simulink model "CANTXcommunicationunit_4"  (R2024a)
settings: Solver=VariableStepAuto  StartTime=0.0  StopTime=10.0  RelTol=1e-3
undefined symbols (not defined in the file or in its folder): canChannel
libraries: canlib x3, canmsglib x2
settings Model: DataDictionary=BMS_System_dict1.sldd  Creator=hirah  LastModifiedBy=hirah

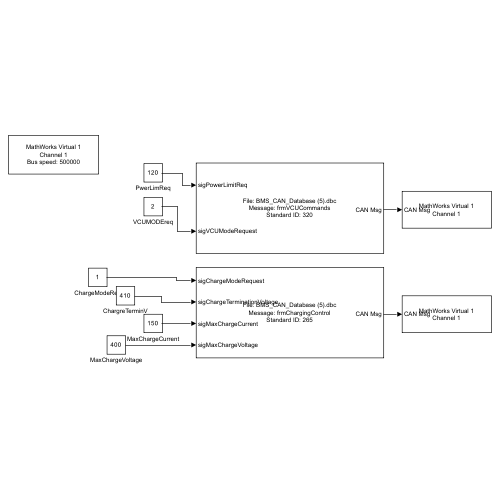
[thumbnail: Simulink's stored preview of the top-level diagram]
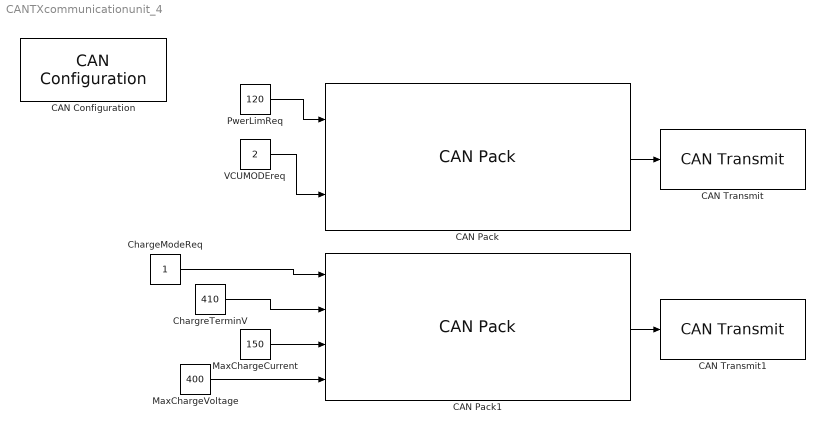
== system CANTXcommunicationunit_4 ==
  CAN Configuration : canlib/CAN Configuration  BlockHandle=708.0002  Device=MathWorks Virtual 1 (Channel 1)  DeviceMenu=MathWorks Virtual 1 (Channel 1)  ObjConstructor=canChannel('MathWorks', 'Virtual 1', 1)  BusSpeed=500000  EnableBitParameters=off  AckMode=Normal
  CAN Pack : canmsglib/CAN Pack  CANdbFile=C:\Users\hirah\Downloads\BMS_CAN_Database (5).dbc  MsgList=frmVCUCommands  MsgName=frmVCUCommands  MsgIDType=Standard (11-bit identifier)  MsgIdentifier=320  MsgLength=3  Remote=off  ApplyMinMax=off  BusOutput=off  SignalInfo={'sigPowerLimitReq','8','16','LE','unsigned','Standard','0','1','0','0','200';'sigVCUModeRequest','0','8','LE','unsigned','Standard','0','1','0','0','5'}
      settings: LibrarySourceBlock=canlib/CAN Pack  DataFormat=CANdb specified signals
  CAN Pack1 : canmsglib/CAN Pack  CANdbFile=C:\Users\hirah\Downloads\BMS_CAN_Database (5).dbc  MsgList=frmChargingControl  MsgName=frmChargingControl  MsgIDType=Standard (11-bit identifier)  MsgIdentifier=265  MsgLength=7  Remote=off  ApplyMinMax=off  BusOutput=off  SignalInfo={'sigChargeModeRequest','48','8','LE','unsigned','Standard','0','1','0','0','3';'sigChargeTerminationVoltage','32','16','LE','unsigned','Standard','0','0.1','0','0','1000';'sigMaxChargeCurrent','16','16','LE','unsigned','Standard','0','0.1','0','0','400';'sigMaxChargeVoltage','0','16','LE','unsigned','Standard','0','0.1','0','0','1000'}
      settings: LibrarySourceBlock=canlib/CAN Pack  DataFormat=CANdb specified signals
  CAN Transmit : canlib/CAN Transmit  BlockHandle=714.0001  Device=MathWorks Virtual 1 (Channel 1)  DeviceMenu=MathWorks Virtual 1 (Channel 1)  ObjConstructor=canChannel('MathWorks', 'Virtual 1', 1)  EnableEventTransmit=off  EnablePeriodicTransmit=off  MessagePeriod=1.000
  CAN Transmit1 : canlib/CAN Transmit  BlockHandle=714.0001  Device=MathWorks Virtual 1 (Channel 1)  DeviceMenu=MathWorks Virtual 1 (Channel 1)  ObjConstructor=canChannel('MathWorks', 'Virtual 1', 1)  EnableEventTransmit=off  EnablePeriodicTransmit=off  MessagePeriod=1.000
  ChargeModeReq : Constant  OutDataTypeStr=uint8
  ChargreTerminV : Constant  Value=410  OutDataTypeStr=double
  MaxChargeCurrent : Constant  Value=150  OutDataTypeStr=double
  MaxChargeVoltage : Constant  Value=400  OutDataTypeStr=double
  PwerLimReq : Constant  Value=120  OutDataTypeStr=uint16
  VCUMODEreq : Constant  Value=2  OutDataTypeStr=uint8
  wires:
  PwerLimReq/1 -> CAN Pack/1
  CAN Pack/1 -> CAN Transmit/1
  VCUMODEreq/1 -> CAN Pack/2
  CAN Pack1/1 -> CAN Transmit1/1
  ChargeModeReq/1 -> CAN Pack1/1
  ChargreTerminV/1 -> CAN Pack1/2
  MaxChargeCurrent/1 -> CAN Pack1/3
  MaxChargeVoltage/1 -> CAN Pack1/4
